simulink library "asbCubeSatEnvironmentLib"  (R2026a)
settings: Solver=VariableStepAuto
undefined symbols (not defined in the file): CubeSatTimeStep, initCond
libraries: sharedutil x3, aerolibconvert2 x1
settings Model: Creator=The MathWorks, Inc.  LastModifiedBy=The MathWorks, Inc.

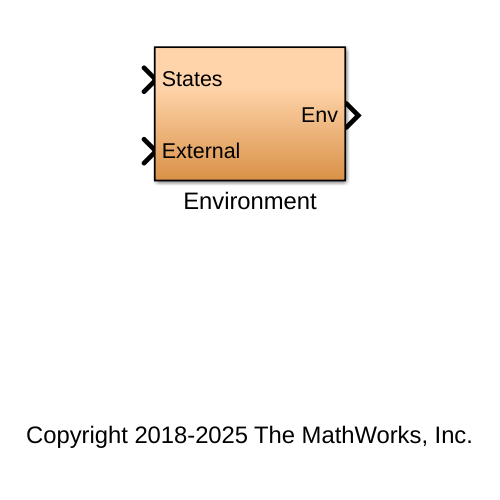
[thumbnail: Simulink's stored preview of the top-level diagram]
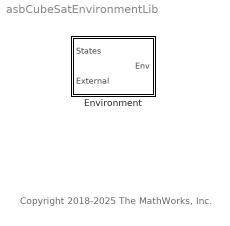
== system asbCubeSatEnvironmentLib ==
  note: Copyright 2018-2025 The MathWorks, Inc.
  Environment : Subsystem  RequirementInfo={} %GIDa_1ba82542_57ba_4b80_8f83_0a428ee4bc68

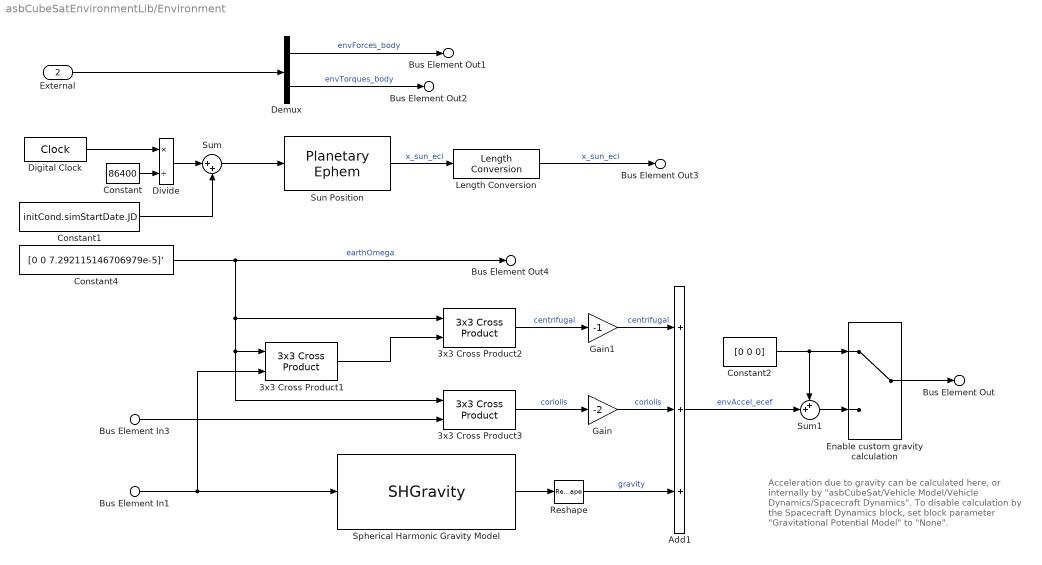
== system asbCubeSatEnvironmentLib/Environment ==
  note: Acceleration due to gravity can be calculated here, or internally by "asbCubeSat/Vehicle Model/Vehicle Dynamics/Spacecraft Dynamics". To disable calculation by the Spacecraft Dynamics block, set block parameter "Gravitational Potential Model" to "None".
  Bus Element In1 : Inport  PortName=States  Element=X_ecef
  Bus Element In3 : Inport  PortName=States  Element=V_ecef
  External : Inport  RequirementInfo={} %GIDa_966e36cb_16b5_4872_900e_7ca1bd630c23  Port=2
  3x3 Cross Product1 : sharedutil/3x3 Cross Product  aMode=aMode
  3x3 Cross Product2 : sharedutil/3x3 Cross Product  aMode=aMode
  3x3 Cross Product3 : sharedutil/3x3 Cross Product  aMode=aMode
  Add1 : Sum  RequirementInfo={} %GIDa_b8d2c483_28a5_4509_a823_93e900185cc4  Inputs=+++
  Constant : Constant  Value=86400
  Constant1 : Constant  RequirementInfo={} %GIDa_d3dce1ea_7a4c_4489_9b49_860fce94c68a  Value=initCond.simStartDate.JD
  Constant2 : Constant  RequirementInfo={} %GIDa_bd077cfd_f306_41c3_b781_8f19467a1c05  Value=[0 0 0]
  Constant4 : Constant  Value=[0 0 7.292115146706979e-5]'
  Demux : Demux  RequirementInfo={} %GIDa_25e02362_af2f_4200_81e6_6d7271b48bfe  Outputs=2
  Digital Clock : DigitalClock  SampleTime=CubeSatTimeStep
  Divide : Product  Inputs=*/
  Enable custom gravity calculation : ManualSwitch
  Gain : Gain  Gain=-2
  Gain1 : Gain  Gain=-1
  Length Conversion : aerolibconvert2/Length Conversion  IU=km  OU=m
  Reshape : Reshape
  Spherical Harmonic Gravity Model : SHGravity  RequirementInfo={} %GIDa_e6b23945_77d7_4eed_b23b_331bed44acc0  degree=20  datafile='aerogmm2b.mat'
  Sum : Sum  Inputs=|++
  Sum1 : Sum  Inputs=++|
  Sun Position : PlanetaryEphem  ephemerisModel=DE421  target=Sun  outputVelocity=off
  Bus Element Out : Outport  VectorParamsAs1DForOutWhenUnconnected=off  PortName=Env  Element=envAccel_ecef
  Bus Element Out1 : Outport  VectorParamsAs1DForOutWhenUnconnected=off  PortName=Env  Element=envForces_body
  Bus Element Out2 : Outport  VectorParamsAs1DForOutWhenUnconnected=off  PortName=Env  Element=envTorques_body
  Bus Element Out3 : Outport  VectorParamsAs1DForOutWhenUnconnected=off  PortName=Env  Element=x_sun_eci
  Bus Element Out4 : Outport  VectorParamsAs1DForOutWhenUnconnected=off  PortName=Env  Element=earthAngRate
  wires:
  Bus Element In1/1 -> 3x3 Cross Product1/2, Spherical Harmonic Gravity Model/1
  Demux/1 -> Bus Element Out1/1  "envForces_body"
  Add1/1 -> Sum1/2  "envAccel_ecef"
  Demux/2 -> Bus Element Out2/1  "envTorques_body"
  External/1 -> Demux/1
  Spherical Harmonic Gravity Model/1 -> Reshape/1
  Sum/1 -> Sun Position/1
  Digital Clock/1 -> Divide/1
  Sun Position/1 -> Length Conversion/1  "x_sun_eci"
  Constant4/1 -> Bus Element Out4/1, 3x3 Cross Product3/1, 3x3 Cross Product1/1, 3x3 Cross Product2/1  "earthOmega"
  Length Conversion/1 -> Bus Element Out3/1  "x_sun_eci"
  Constant/1 -> Divide/2
  Divide/1 -> Sum/1
  Constant1/1 -> Sum/2
  Reshape/1 -> Add1/3  "gravity"
  3x3 Cross Product1/1 -> 3x3 Cross Product2/2
  Bus Element In3/1 -> 3x3 Cross Product3/2
  3x3 Cross Product3/1 -> Gain/1  "coriolis"
  3x3 Cross Product2/1 -> Gain1/1  "centrifugal"
  Gain1/1 -> Add1/1  "centrifugal"
  Gain/1 -> Add1/2  "coriolis"
  Constant2/1 -> Sum1/1, Enable custom gravity calculation/1
  Enable custom gravity calculation/1 -> Bus Element Out/1
  Sum1/1 -> Enable custom gravity calculation/2
